simulink model "rlsfiltersystemidentification"  (R2014a)
settings: Solver=FixedStepDiscrete  StartTime=0.0  StopTime=Inf  RelTol=1e-3
InitFcn:
  | Ts = 1/44.1e3;
  | L = 1024;
values from neighbouring files (symbols this model uses):
  F = 75    [HelperAdaptiveNoiseCancellation.m]
libraries: dspmathops x2, dspsrcs4 x1, dspswit3 x1, dspadpt3 x1, dspspect3 x1, dspsnks4 x1
CloseFcn:
  | clear Ts L
  | close all force
settings Model: Creator=The MathWorks Inc.
settings DebuggingCC: UnderspecifiedInitializationDetection=Classic

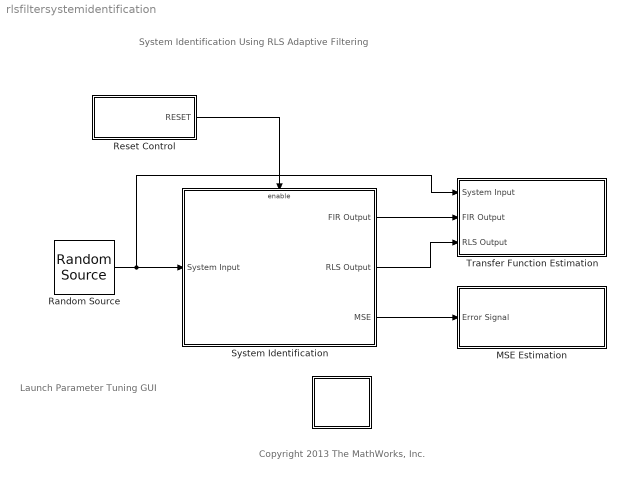
== system rlsfiltersystemidentification ==
  note: Launch Parameter Tuning GUI
  note: Copyright 2013 The MathWorks, Inc.
  note: System Identification Using RLS Adaptive Filtering
  " " : Subsystem  TreatAsAtomicUnit=on
      settings: OpenFcn=web(fullfile(matlabroot,'toolbox','dsp','dspdemos','html','RLSFilterSystemIdentificationExample.html'),'-helpbrowser')
      mask Display: disp('info')
  MSE Estimation : Subsystem  TreatAsAtomicUnit=on
  Random Source : dspsrcs4/Random Source  SrcType=Gaussian  NormMethod=Ziggurat  CltLength=12  MinVal=0  MaxVal=1  MeanVal=0  VarVal=1e-2  RepMode=Specify seed  rawSeed=1  IsInherit=off  SampMode=Discrete  SampTime=Ts  SampFrame=L  DataType=Double  OutComplex=Real
  Reset Control : Subsystem
  System Identification : Subsystem  TreatAsAtomicUnit=on
  Transfer Function Estimation : Subsystem  TreatAsAtomicUnit=on
  wires:
  Random Source/1 -> Transfer Function Estimation/1(System Input), System Identification/1(System Input)
  Reset Control/1(RESET) -> System Identification/Enable
  System Identification/3(MSE) -> MSE Estimation/1(Error Signal)
  System Identification/2(RLS Output) -> Transfer Function Estimation/3(RLS Output)
  System Identification/1(FIR Output) -> Transfer Function Estimation/2(FIR Output)

== system rlsfiltersystemidentification/  ==

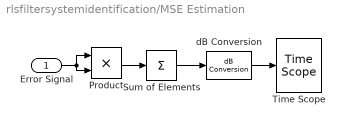
== system rlsfiltersystemidentification/MSE Estimation ==
  Error Signal : Inport
  Product : Product
  Sum of Elements : Sum  Inputs=+
  Time Scope : TimeScope  DefaultConfigurationName=spbscopes.TimeScopeBlockCfg
  dB Conversion : dspmathops/dB Conversion  dBtype=dB  intype=Amplitude  R=1  fuzz=on
  wires:
  dB Conversion/1 -> Time Scope/1
  Error Signal/1 -> Product/1, Product/2
  Product/1 -> Sum of Elements/1
  Sum of Elements/1 -> dB Conversion/1

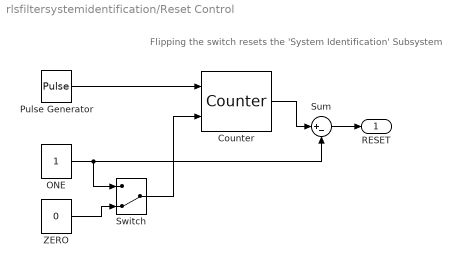
== system rlsfiltersystemidentification/Reset Control ==
  note: Flipping the switch resets the 'System Identification' Subsystem
  Counter : dspswit3/Counter  Direction=Up  CountEvent=Either edge  CounterSize=32 bits  MaxCount=1  InitialCount=0  Output=Count  HitValue=32  ResetInput=on  SamplesPerFrame=1  Ts=Ts * F  CntDtype=double  HitDtype=Logical
  ONE : Constant  VectorParams1D=off
  Pulse Generator : DiscretePulseGenerator  SampleTime=Ts * L
  Sum : Sum  Inputs=|+-
  Switch : ManualSwitch  CurrentSetting=0
  ZERO : Constant  Value=0  VectorParams1D=off
  RESET : Outport
  wires:
  Counter/1 -> Sum/1
  Pulse Generator/1 -> Counter/1
  ZERO/1 -> Switch/2
  Sum/1 -> RESET/1
  Switch/1 -> Counter/2
  ONE/1 -> Sum/2, Switch/1

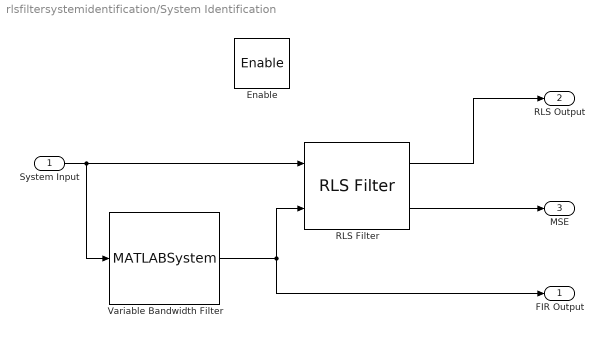
== system rlsfiltersystemidentification/System Identification ==
  System Input : Inport
  Enable : EnablePort  StatesWhenEnabling=reset
  RLS Filter : dspadpt3/RLS Filter  L=29  lambdaflag=Dialog  lambda=0.99  addnparflag=on  ic=0  delta=0.1  Adapt=off  resetflag=None  weights=off
  Variable Bandwidth Filter : MATLABSystem  System=dsp.VariableBandwidthFIRFilter  SampleRate=1/Ts  FilterOrder=30  FilterType=Lowpass  CutoffFrequency=5000  CenterFrequency=44100/4  Bandwidth=7680  Window=Kaiser  KaiserWindowParameter=8  SidelobeAttenuation=60
      mask Type: dsp.VariableBandwidthFIRFilter
      mask Display:
      | disp(['Variable Bandwidth' char(10) 'FIR Filter']);
      | port_label('input',1,'x');
      | port_label('output',1,'y');
  FIR Output : Outport
  RLS Output : Outport  Port=2
  MSE : Outport  Port=3
  wires:
  System Input/1 -> Variable Bandwidth Filter/1, RLS Filter/1
  Variable Bandwidth Filter/1 -> FIR Output/1, RLS Filter/2
  RLS Filter/1 -> RLS Output/1
  RLS Filter/2 -> MSE/1

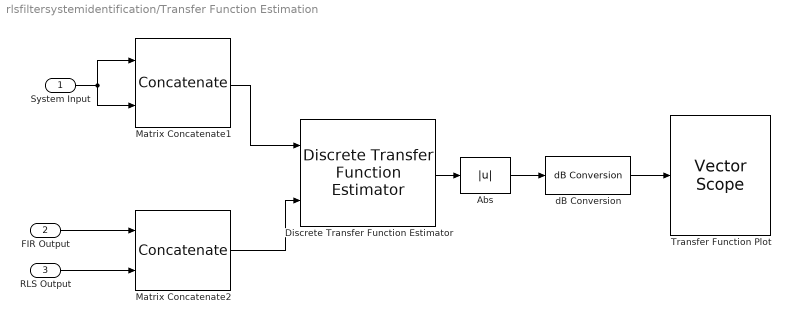
== system rlsfiltersystemidentification/Transfer Function Estimation ==
  System Input : Inport
  FIR Output : Inport  Port=2
  RLS Output : Inport  Port=3
  Abs : Abs
  Discrete Transfer Function Estimator : dspspect3/Discrete Transfer Function Estimator  SimulateUsing=Code generation  SpectralAverages=5  FFTLengthSource=Auto  FFTLength=128  Window=Hann  SidelobeAttenuation=60  FrequencyRange=onesided
  Matrix Concatenate1 : Concatenate  Mode=Multidimensional array  ConcatenateDimension=2
  Matrix Concatenate2 : Concatenate  Mode=Multidimensional array  ConcatenateDimension=2
  "Transfer Function Plot " : dspsnks4/Vector Scope  ScopeProperties=on  Domain=User-defined  HorizSpan=1  DisplayProperties=off  AxisGrid=on  Memory=off  FrameNumber=off  AxisLegend=on  AxisZoom=off  OpenScopeAtSimStart=on  OpenScopeImmediately=off  FigPos=[400 205 398 313]  AxisProperties=off  XUnits=Hertz  XRange=[0...Fs/2]  InheritXIncr=off  XIncr=.5 * 44.1*1e3/513  XLabel=Frequency (Hz)  XLimit=Auto  XMin=0  XMax=1  XStart=0  YUnits=dB  YLabel=Amplitude (dB)  LineProperties=off  LineStyles=-  LineMarkers=None  LineColors=[0 0 1]|[1 0 0]  XAxisParamsVer=6.9
      settings: YMin=-80  YMax=1
  dB Conversion : dspmathops/dB Conversion  dBtype=dB  intype=Amplitude  R=1  fuzz=on
  wires:
  Matrix Concatenate2/1 -> Discrete Transfer Function Estimator/2
  Discrete Transfer Function Estimator/1 -> Abs/1
  FIR Output/1 -> Matrix Concatenate2/1
  RLS Output/1 -> Matrix Concatenate2/2
  Matrix Concatenate1/1 -> Discrete Transfer Function Estimator/1
  dB Conversion/1 -> "Transfer Function Plot "/1
  Abs/1 -> dB Conversion/1
  System Input/1 -> Matrix Concatenate1/2, Matrix Concatenate1/1
